simulink model "pct23_P_reg"  (R2020b)
settings: Solver=FixedStepAuto  StartTime=0.0  StopTime=12000  FixedStep=Ts  RelTol=1e-3
values from neighbouring files (symbols this model uses):
  Ts = 0.5    [mpc_init_reference_tracking.m]    (also in pct23_init.m; ref_tracking21.mat; ref_tracking25.mat; ref_tracking26.mat)
libraries: pid_lib x1, pct23_lib x1
settings Model: Creator=belko  LastModifiedBy=lgalc

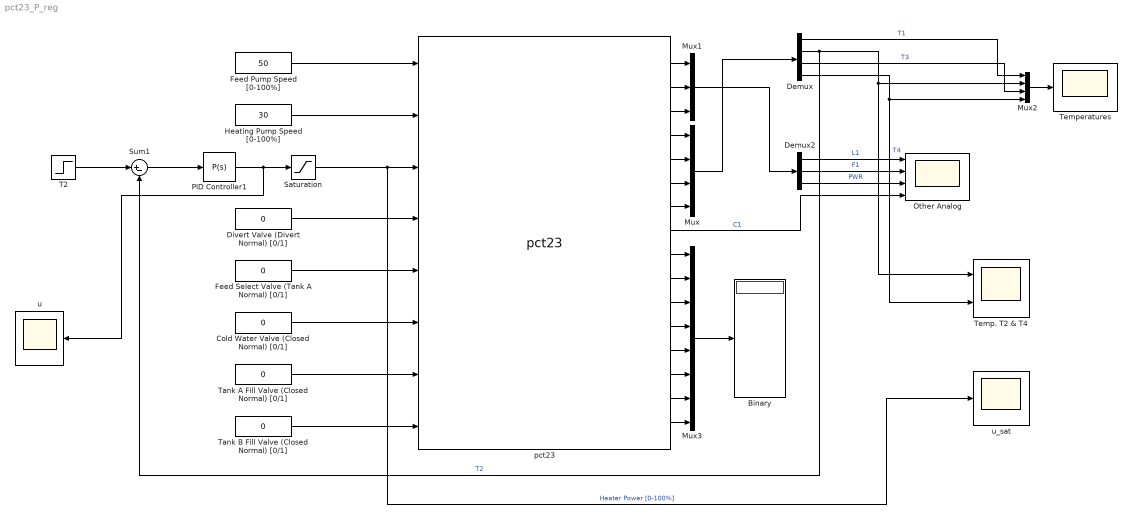
== system pct23_P_reg ==
  Binary : Display
  Cold Water Valve (Closed Normal) [0/1] : Constant  Value=0
  Demux : Demux
  Demux2 : Demux  Outputs=3
  Divert Valve (Divert Normal) [0/1] : Constant  Value=0
  Feed Pump Speed [0-100%] : Constant  Value=50
  Feed Select Valve (Tank A Normal) [0/1] : Constant  Value=0
  Heating Pump Speed [0-100%] : Constant  Value=30
  Mux : Mux
  Mux1 : Mux  Inputs=3
  Mux2 : Mux
  Mux3 : Mux  Inputs=8
  Other Analog : Scope  NumInputPorts=4
  PID Controller1 : pid_lib/PID Controller  Controller=P  Form=Parallel  TimeDomain=Continuous-time  UseExternalTs=off  SampleTime=Ts  IntegratorMethod=Forward Euler  FilterMethod=Forward Euler  ControllerParametersSource=internal  P=20  I=1  D=0  UseFilter=on  N=100  TunerSelectOption=Transfer Function Based (PID Tuner App)  InitialConditionSource=internal  InitialConditionForIntegrator=0  InitialConditionForFilter=0  DifferentiatorICPrevScaledInput=0  ExternalReset=none  TrackingMode=off  Kt=1  LimitOutput=off  SatLimitsSource=internal  UpperSaturationLimit=inf  LowerSaturationLimit=-inf  LinearizeAsGain=on  AntiWindupMode=none  Kb=1  POutMin=[]  POutMax=[]  IOutMin=[]  IOutMax=[]  DOutMin=[]  DOutMax=[]  NOutMin=[]  NOutMax=[]  SumOutMin=[]  SumOutMax=[]  SaturationOutMin=[]  SaturationOutMax=[]  PParamMin=[]  PParamMax=[]  IParamMin=[]  IParamMax=[]  DParamMin=[]  DParamMax=[]  NParamMin=[]  NParamMax=[]  KbParamMin=[]  KbParamMax=[]  KtParamMin=[]  KtParamMax=[]  KbOutMin=[]  KbOutMax=[]  KtOutMin=[]  KtOutMax=[]  IntegratorOutMin=[]  IntegratorOutMax=[]  FilterOutMin=[]  FilterOutMax=[]  SumI1OutMin=[]  SumI1OutMax=[]  SumI2OutMin=[]  SumI2OutMax=[]  SumI3OutMin=[]  SumI3OutMax=[]  SumI4OutMin=[]  SumI4OutMax=[]  SumDOutMin=[]  SumDOutMax=[]  DifferentiatorOutMin=[]  DifferentiatorOutMax=[]  FilterDiffOutCoefMin=[]  FilterDiffOutCoefMax=[]  ReciprocalOutMin=[]  ReciprocalOutMax=[]  SumDenOutMin=[]  SumDenOutMax=[]  SumNumOutMin=[]  SumNumOutMax=[]  DivideOutMin=[]  DivideOutMax=[]  UdiffTsProdOutMin=[]  UdiffTsProdOutMax=[]  NTsProdOutMin=[]  NTsProdOutMax=[]  UintegralTsProdOutMin=[]  UintegralTsProdOutMax=[]  UngainTsProdOutMin=[]  UngainTsProdOutMax=[]  IntegratorContinuousStateAttributes=''  IntegratorStateMustResolveToSignalObject=off  IntegratorRTWStateStorageClass=Auto  FilterContinuousStateAttributes=''  FilterStateMustResolveToSignalObject=off  FilterRTWStateStorageClass=Auto  ParallelPVariant=InternalParameters  IdealPVariant=Disabled  IVariant=Disabled  DVariant=Disabled  IntegratorVariant=Disabled  SatVariant=Disabled  AWVariant=Disabled  PCopyVariant=Disabled  TRVariant=Disabled  FdbkBlocksVariant=Forward  IdealPFdbkVariant=Disabled  SatFdbkVariant=Disabled  DerivativeFilterVariant=Disabled  NVariant=Disabled  NCopyVariant=Disabled_SignalSpec  FilterICVariant=Disabled  IntegratorICVariant=Disabled  ExternalResetVariant=Disabled  TRSumVariant=Passthrough  SumFdbkVariant=Disabled  SumVariant=Passthrough_P  TsampFilterVariant=InternalTs  TsampNgainVariant=Passthrough  TsampIntegralVariant=Disabled_SignalSpec  ExternalSaturationOutDataTypeStr=Inherit: Same as second input
  Saturation : Saturate  UpperLimit=100  LowerLimit=0
  Sum1 : Sum  Inputs=|+-
  T2 : Step  Time=0  Before=71  After=71  SampleTime=0
  Tank A Fill Valve (Closed Normal) [0/1] : Constant  Value=0
  Tank B Fill Valve (Closed Normal) [0/1] : Constant  Value=0
  Temp. T2 & T4 : Scope  NumInputPorts=2
  Temperatures : Scope
  pct23 : pct23_lib/pct23  SystemSampleTime=-1  VariantActivationTime=update diagram  Latency=0  AutoFrameSizeCalculation=off
  u : Scope
  u_sat : Scope
  wires:
  PID Controller1/1 -> u/1, Saturation/1
  Saturation/1 -> u_sat/1, pct23/3  "Heater Power [0-100%]"
  Mux3/1 -> Binary/1
  pct23/3 -> Mux1/3
  Sum1/1 -> PID Controller1/1
  T2/1 -> Sum1/1
  Demux/2 -> Temp. T2 & T4/1, Mux2/2, Sum1/2  "T2"
  pct23/15 -> Mux3/7
  Heating Pump Speed [0-100%]/1 -> pct23/2
  pct23/9 -> Mux3/1
  Mux1/1 -> Demux2/1
  Demux2/3 -> Other Analog/3  "PWR"
  pct23/11 -> Mux3/3
  pct23/2 -> Mux1/2
  pct23/14 -> Mux3/6
  pct23/8 -> Other Analog/4  "C1"
  pct23/10 -> Mux3/2
  Demux/3 -> Mux2/3  "T3"
  pct23/6 -> Mux/3
  Demux/1 -> Mux2/1  "T1"
  Feed Select Valve (Tank A Normal) [0/1]/1 -> pct23/5
  pct23/16 -> Mux3/8
  pct23/1 -> Mux1/1
  Divert Valve (Divert Normal) [0/1]/1 -> pct23/4
  pct23/5 -> Mux/2
  pct23/4 -> Mux/1
  Demux2/2 -> Other Analog/2  "F1"
  Demux2/1 -> Other Analog/1  "L1"
  pct23/13 -> Mux3/5
  pct23/7 -> Mux/4
  Tank B Fill Valve (Closed Normal) [0/1]/1 -> pct23/8
  pct23/12 -> Mux3/4
  Cold Water Valve (Closed Normal) [0/1]/1 -> pct23/6
  Demux/4 -> Mux2/4, Temp. T2 & T4/2  "T4"
  Mux/1 -> Demux/1
  Feed Pump Speed [0-100%]/1 -> pct23/1
  Tank A Fill Valve (Closed Normal) [0/1]/1 -> pct23/7
  Mux2/1 -> Temperatures/1
